simulink model "singleph_invload"  (R2017b)
settings: Solver=ode23t  StartTime=0.0  StopTime=1  MinStep=1e-6  RelTol=1e-3
libraries: powerlib x17
settings Model: Creator=VMORAIS  LastModifiedBy=VMORAIS

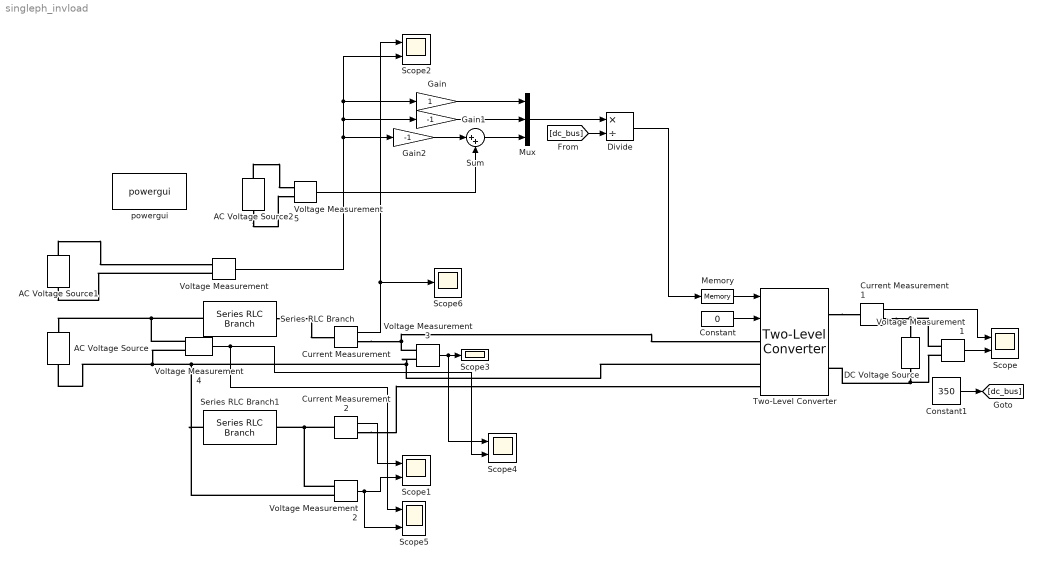
== system singleph_invload ==
  AC Voltage Source : powerlib/Electrical Sources/AC Voltage Source  Amplitude=325  Phase=0  Frequency=50  SampleTime=0  Measurements=None  BusType=swing  Pref=10e3  Qref=0  Qmin=-inf  Qmax=+inf
  AC Voltage Source1 : powerlib/Electrical Sources/AC Voltage Source  Amplitude=325  Phase=0.2  Frequency=50  SampleTime=0  Measurements=None  BusType=swing  Pref=10e3  Qref=0  Qmin=-inf  Qmax=+inf
  AC Voltage Source2 : powerlib/Electrical Sources/AC Voltage Source  Amplitude=50  Phase=0  Frequency=10  SampleTime=0  Measurements=None  BusType=swing  Pref=10e3  Qref=0  Qmin=-inf  Qmax=+inf
  Constant : Constant  Value=0
  Constant1 : Constant  Value=350
  Current Measurement : powerlib/Measurements/Current Measurement  PhasorSimulation=off  OutputType=Complex  PSBequivalent=0
  Current Measurement1 : powerlib/Measurements/Current Measurement  PhasorSimulation=off  OutputType=Complex  PSBequivalent=0
  Current Measurement2 : powerlib/Measurements/Current Measurement  PhasorSimulation=off  OutputType=Complex  PSBequivalent=0
  DC Voltage Source : powerlib/Electrical Sources/DC Voltage Source  Amplitude=350  Measurements=None
  Divide : Product  Inputs=*/
  Gain : Gain
  Gain1 : Gain  Gain=-1
  Gain2 : Gain  Gain=-1
  Memory : Memory
  Mux : Mux  Inputs=3
  Scope{,1..2,4..5} (5 alike) : Scope  NumInputPorts=2
  Scope3 : Scope
  Scope6 : Scope
  Series RLC Branch : powerlib/Elements/Series RLC Branch  LConnTagsString=__new0  RConnTagsString=__new0  BranchType=RL  Resistance=1e-2  Inductance=1e-3  SetiL0=on  InitialCurrent=0  Capacitance=1e-6  Setx0=off  InitialVoltage=0  Measurements=None
  Series RLC Branch1 : powerlib/Elements/Series RLC Branch  LConnTagsString=__new0  RConnTagsString=__new0  BranchType=R  Resistance=10  Inductance=1e-2  SetiL0=off  InitialCurrent=0  Capacitance=1e-6  Setx0=off  InitialVoltage=0  Measurements=None
  Sum : Sum  Inputs=|++
  Two-Level Converter : powerlib/Power Electronics/Two-Level Converter  ModelType=Average model (Uref-controlled)  Ron=1e-3  Rs=1e6  Cs=inf  Vforward=[0,0]  Ron_Diode=1e-3  Rs_Diode=1e6  Cs_Diode=inf  Vf_Diode=1e-3  Rs_CurrentSource=inf
      settings: SourceProductName=Simscape Power Systems  SourceProductBaseCode=PS
  Voltage Measurement{,1..5} (6 alike) : powerlib/Measurements/Voltage Measurement  PhasorSimulation=off  OutputType=Complex  PSBequivalent=0
  powergui : powerlib/powergui  Priority=1  SimulationMode=Continuous  SampleTime=50e-6  frequency=60  Iterations=50  frequencyindice=10  Pbase=100e6  ErrMax=1e-4  UnitsV=kV  UnitsW=MW  buscounter=0  FunctionMessages=off  echomessages=off  EnableUseOfTLC=off  CurrentSourceSwitches=off  DisableSnubberDevices=off  DisableRonSwitches=off  DisableVfSwitches=off  DisplayEquations=off  SolverType=Tustin/Backward Euler (TBE)  Interpol=off  ExternalGateDelay=off  methode=off  Ts=100  x0status=blocks  SPID=on  SwTol=0  HookPort=off  RestoreLinks=warning  ResistiveCurrentMeasurement=off  Frange=[0:2:500]  Ylog=off  Xlog=on  ShowGrid=off  save=off  variable=ZData  structure=0  ZoomFFT=off  StartTime=0.0  cycles=1  DisplayStyle=1  fundamental=60  FreqAxis=off  MaxFrequency=1000  frequencyindicesteady=1  RmsSteady=1  display=off
  wires:
  Constant/1 -> Two-Level Converter/2
  Voltage Measurement1/1 -> Scope/2
  Current Measurement1/1 -> Scope/1
  Mux/1 -> Divide/1
  Gain/1 -> Mux/1
  Memory/1 -> Two-Level Converter/1
  Gain1/1 -> Mux/2
  Voltage Measurement/1 -> Scope2/2, Gain/1, Gain1/1, Gain2/1
  Gain2/1 -> Sum/1
  Current Measurement2/1 -> Scope1/1
  Voltage Measurement2/1 -> Scope5/2, Scope1/2
  Current Measurement/1 -> Scope6/1, Scope2/1
  Voltage Measurement3/1 -> Scope4/1, Scope3/1
  [dc_bus] -> Divide/2
  Divide/1 -> Memory/1
  Constant1/1 -> [dc_bus]
  Voltage Measurement4/1 -> Scope5/1, Scope4/2
  Sum/1 -> Mux/3
  Voltage Measurement5/1 -> Sum/2
  connections:
  Two-Level Converter/LConn2 -- Voltage Measurement3/LConn2 -- Voltage Measurement2/LConn2 -- Series RLC Branch1/LConn1 -- Voltage Measurement4/LConn2 -- AC Voltage Source/LConn1
  Series RLC Branch/LConn1 -- Voltage Measurement4/LConn1 -- AC Voltage Source/RConn1
  DC Voltage Source/LConn1 -- Voltage Measurement1/LConn2 -- Two-Level Converter/RConn2
  Two-Level Converter/RConn1 -- Current Measurement1/LConn1
  Series RLC Branch/RConn1 -- Current Measurement/LConn1
  Current Measurement2/RConn1 -- Two-Level Converter/LConn3
  Current Measurement/RConn1 -- Voltage Measurement3/LConn1 -- Two-Level Converter/LConn1
  Current Measurement1/RConn1 -- Voltage Measurement1/LConn1 -- DC Voltage Source/RConn1
  Current Measurement2/LConn1 -- Voltage Measurement2/LConn1 -- Series RLC Branch1/RConn1
  AC Voltage Source1/RConn1 -- Voltage Measurement/LConn1
  Voltage Measurement/LConn2 -- AC Voltage Source1/LConn1
  AC Voltage Source2/RConn1 -- Voltage Measurement5/LConn1
  AC Voltage Source2/LConn1 -- Voltage Measurement5/LConn2
